simulink model "trial_lecture_Simulator_TeppoLuukkonen"  (R2024a)
settings: Solver=VariableStepAuto  StartTime=0.0  StopTime=6  RelTol=1e-3
values from neighbouring files (symbols this model uses):
  g = 9.81    [trial_lecture_settings.m]
  gamma = k_M / k_F    (= 0.0301068588469)    [trial_lecture_settings.m]
  I = diag([Ixx Iyy Izz])    [trial_lecture_settings.m]
  L = 0.1785    [trial_lecture_settings.m]
  m = 0.429    [trial_lecture_settings.m]
  rz = 5    [trial_lecture_settings.m]
libraries: vrlib x1, sharedtransform x1, uavutilslib x1
settings Model: PacingRate=0.800000  Creator=ZHE SHEN  LastModifiedBy=lucid
settings SolverCC: AlgebraicLoopSolver=TrustRegion
settings DebuggingCC: UnconnectedInputMsg=warning  UnconnectedOutputMsg=warning  UnconnectedLineMsg=warning  UnderSpecifiedDimensionMsg=warning
settings ModelReferenceCC: EnableRefExpFcnMdlSchedulingChecks=on
settings RTWCC: GPUComputeCapability=3.5  DLArmComputeVersion=19.05

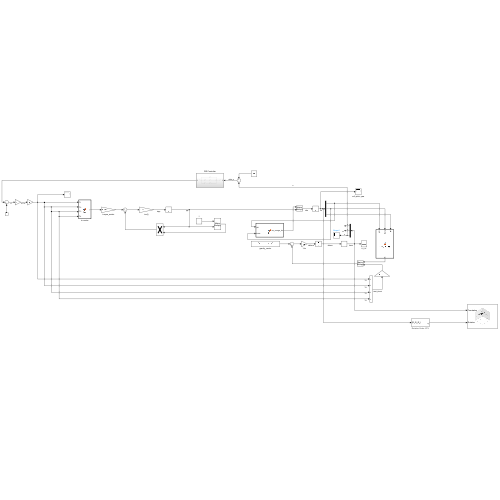
[thumbnail: Simulink's stored preview of the top-level diagram]
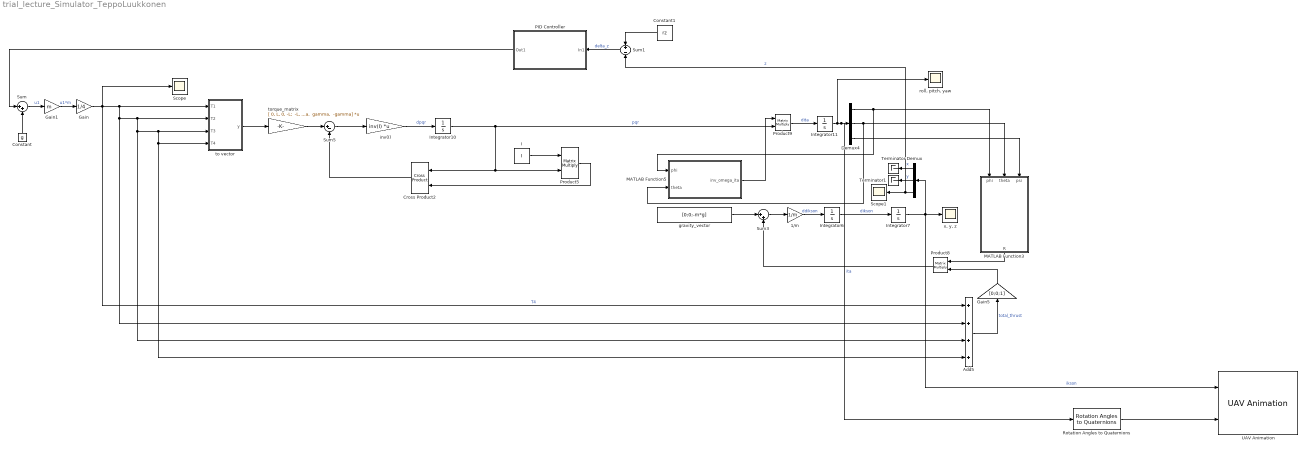
== system trial_lecture_Simulator_TeppoLuukkonen ==
  1/m : Gain  Gain=1/m
  Add5 : Sum  Inputs=++++
  Constant : Constant  Value=g
  Constant1 : Constant  Value=rz
  Cross Product2 : vrlib/Utilities/Cross Product
  Demux : Demux  Outputs=3
  Demux4 : Demux  Outputs=3
  Gain : Gain  Gain=1/4
  Gain1 : Gain  Gain=m
  Gain5 : Gain  Gain=[0;0;1]
  I : Constant  Value=I
  Integrator{6..7,10..11} (4 alike) : Integrator
  MATLAB Function3 : MATLAB Function  TreatAsAtomicUnit=on
  MATLAB Function5 : MATLAB Function  TreatAsAtomicUnit=on
  PID Controller : Subsystem
  Product5 : Product  Multiplication=Matrix(*)
  Product8 : Product  Multiplication=Matrix(*)
  Product9 : Product  Multiplication=Matrix(*)
  Rotation Angles to Quaternions : sharedtransform/Rotation Angles to Quaternions  rotationOrder=ZYX  aMode=aMode
  Scope : Scope
  Scope1 : Scope
  Sum : Sum  Inputs=|++
  Sum1 : Sum  Inputs=+|-
  Sum3 : Sum  Inputs=|++
  Sum5 : Sum  Inputs=|+-
  Terminator : Terminator
  Terminator1 : Terminator
  UAV Animation : uavutilslib/UAV Animation  UAVType=Multirotor  UAVSize=1  InertialZDirection=Up  SampleTime=-1
  gravity_vector : Constant  Value=[0;0;-m*g]
  inv(I) : Gain  Gain=inv(I)  Multiplication=Matrix(K*u) (u vector)
  "roll, pitch, yaw" : Scope
  to vector : MATLAB Function  TreatAsAtomicUnit=on
  torque_matrix : Gain  Gain="[ 0, L, 0, -L;  -L, 0,  L,  0; gamma,  -gamma,  gamma,  -gamma]"  Multiplication=Matrix(K*u) (u vector)
  "x, y, z" : Scope
  wires:
  Gain5/1 -> Product8/2
  torque_matrix/1 -> Sum5/1
  Product9/1 -> Integrator11/1  "dita"
  Integrator11/1 -> Rotation Angles to Quaternions/1, Demux4/1, "roll, pitch, yaw"/1  "ita"
  Add5/1 -> Gain5/1  "total_thrust"
  inv(I)/1 -> Integrator10/1  "dpqr"
  Cross Product2/1 -> Sum5/2
  Demux4/2 -> MATLAB Function3/2(theta), MATLAB Function5/2(theta)
  Sum5/1 -> inv(I)/1
  MATLAB Function5/1(inv_omega_ita) -> Product9/1
  Gain/1 -> Scope/1, to vector/4(T4), Add5/4, to vector/3(T3), Add5/3, to vector/2(T2), Add5/2, to vector/1(T1), Add5/1  "T4"
  Integrator6/1 -> Integrator7/1  "dikson"
  Product5/1 -> Cross Product2/2
  Demux4/3 -> MATLAB Function3/3(psi)
  I/1 -> Product5/1
  gravity_vector/1 -> Sum3/1
  Integrator7/1 -> UAV Animation/1, Demux/1, "x, y, z"/1  "ikson"
  Sum3/1 -> 1/m/1
  Demux4/1 -> MATLAB Function3/1(phi), MATLAB Function5/1(phi)
  Product8/1 -> Sum3/2
  Integrator10/1 -> Cross Product2/1, Product5/2, Product9/2  "pqr"
  MATLAB Function3/1(R) -> Product8/1
  1/m/1 -> Integrator6/1  "ddikson"
  to vector/1(y) -> torque_matrix/1
  Gain1/1 -> Gain/1  "u1*m"
  Sum/1 -> Gain1/1  "u1"
  Constant/1 -> Sum/2
  Demux/1 -> Terminator/1  "x"
  Demux/2 -> Terminator1/1  "y"
  Demux/3 -> Scope1/1, Sum1/2  "z"
  Constant1/1 -> Sum1/1
  Sum1/1 -> PID Controller/1(In1)  "delta_z"
  PID Controller/1(Out1) -> Sum/1
  Rotation Angles to Quaternions/1 -> UAV Animation/2

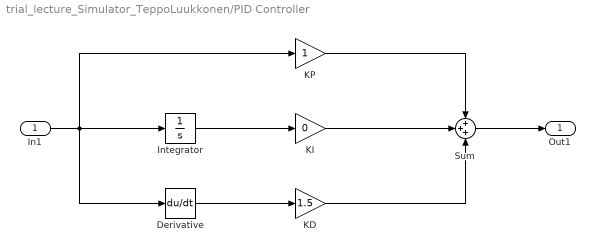
== system trial_lecture_Simulator_TeppoLuukkonen/PID Controller ==
  In1 : Inport
  Derivative : Derivative
  Integrator : Integrator
  KD : Gain  Gain=1.5
  KI : Gain  Gain=0
  KP : Gain
  Sum : Sum  Inputs=+++
  Out1 : Outport
  wires:
  Sum/1 -> Out1/1
  KP/1 -> Sum/1
  KI/1 -> Sum/2
  KD/1 -> Sum/3
  Integrator/1 -> KI/1
  In1/1 -> KP/1, Derivative/1, Integrator/1
  Derivative/1 -> KD/1

== matlab function trial_lecture_Simulator_TeppoLuukkonen/to vector ==
  data: T1 input; y output; T2 input; T3 input; T4 input
function y = fcn(T1,T2,T3,T4)

y = [T1; T2; T3; T4];

== matlab function trial_lecture_Simulator_TeppoLuukkonen/MATLAB Function3 ==
  data: phi input; R output; theta input; psi input
function R = body2inertia(phi,theta,psi)


matrix = [ cos(psi)*cos(theta)   cos(psi)*sin(theta)*sin(phi) -  sin(psi)*cos(phi)   cos(psi)*sin(theta)*cos(phi) +  sin(psi)*sin(phi);
           sin(psi)*cos(theta)   sin(psi)*sin(theta)*sin(phi) +  cos(psi)*cos(phi)   sin(psi)*sin(theta)*cos(phi) -  cos(psi)*sin(phi); 
           -sin(theta)           cos(theta)*sin(phi)                                 cos(theta)*cos(phi) ];



R = matrix;

== matlab function trial_lecture_Simulator_TeppoLuukkonen/MATLAB Function5 ==
  data: phi input; inv_omega_ita output; theta input
function inv_omega_ita = fcn(phi,theta)


matrix = [  1   sin(phi)*tan(theta) cos(phi)*tan(theta);
            0   cos(phi)            -sin(phi);
            0   sin(phi)/cos(theta) cos(phi)/cos(theta)  ];



inv_omega_ita = matrix;
